simulink model "ClosedLoop_CqCscCi"  (R2024a)
settings: Solver=VariableStepAuto  StartTime=0.0  StopTime=10.0  RelTol=1e-3
libraries: RCTblocks x5
settings Model: Creator=Thoma  LastModifiedBy=Thoma

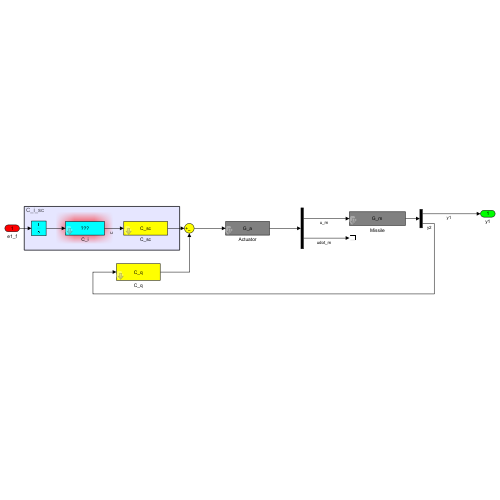
[thumbnail: Simulink's stored preview of the top-level diagram]
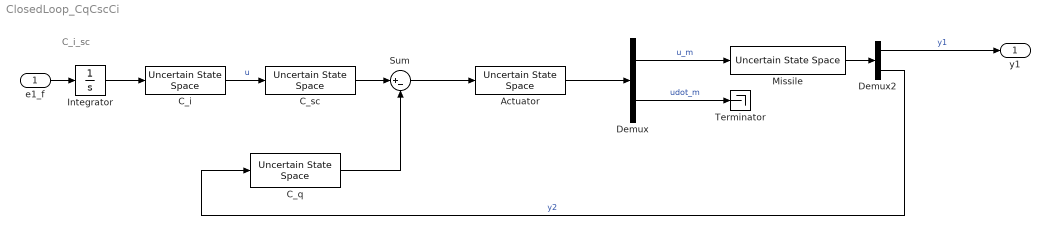
== system ClosedLoop_CqCscCi ==
  note: C_i_sc
  e1_f : Inport
  Actuator : RCTblocks/Uncertain State Space  Tag=USS  USystem=G_a  UValue=[]  X0=[]  uX0=[]
  C_i : RCTblocks/Uncertain State Space  Tag=USS  USystem=C_i  UValue=[]  X0=[]  uX0=[]
  C_q : RCTblocks/Uncertain State Space  Tag=USS  USystem=C_q  UValue=[]  X0=[]  uX0=[]
  C_sc : RCTblocks/Uncertain State Space  Tag=USS  USystem=C_sc  UValue=[]  X0=[]  uX0=[]
  Demux : Demux  Outputs=2
  Demux2 : Demux  Outputs=2
  Integrator : Integrator
  Missile : RCTblocks/Uncertain State Space  Tag=USS  USystem=G_m  UValue=[]  X0=[]  uX0=[]
  Sum : Sum  Inputs=|+-
  Terminator : Terminator
  y1 : Outport
  wires:
  C_sc/1 -> Sum/1
  C_q/1 -> Sum/2
  Missile/1 -> Demux2/1
  Sum/1 -> Actuator/1
  Demux2/1 -> y1/1  "y1"
  Demux/2 -> Terminator/1  "udot_m"
  Actuator/1 -> Demux/1
  Demux2/2 -> C_q/1  "y2"
  Demux/1 -> Missile/1  "u_m"
  e1_f/1 -> Integrator/1
  Integrator/1 -> C_i/1
  C_i/1 -> C_sc/1  "u"
